simulink model "mixed_sensitivity_nonlin"  (R2022b)
settings: Solver=VariableStepAuto  StartTime=0.0  StopTime=1000  RelTol=1e-3
values from neighbouring files (symbols this model uses):
  a = Mv+mp+2*ma+2*IAy/(ra^2)    (= 19.1666666667)    [function_f.m]
  b = 1/2*(Mv*l^2+mp*L^2+2*ma*d^2+IGz+IPz+2*IAz+2*IAy*(d/ra)^2)    (= 3.3525)    [function_f.m]
  IPy = 0.15    [function_f.m]
  IPz = 0.23    [function_f.m]
  L = 1    [function_f.m]
  rp = 0.3    [function_f.m]
undefined symbols (not defined in the file or in its folder): Amix, Bmix, Cmix, Dmix, X_start_lqg_nonlin
settings Model: Creator=franc  LastModifiedBy=Giorgia

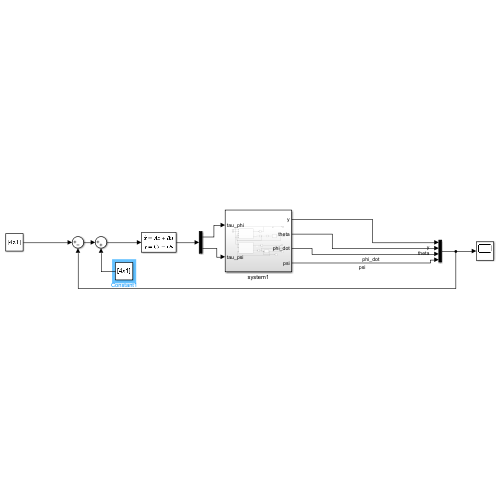
[thumbnail: Simulink's stored preview of the top-level diagram]
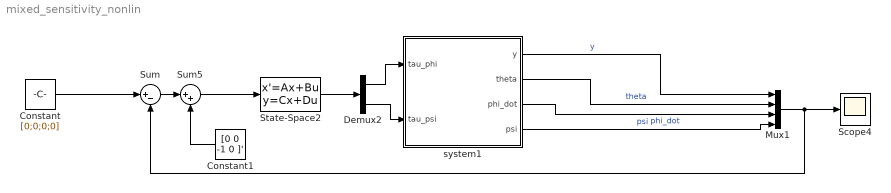
== system mixed_sensitivity_nonlin ==
  Constant : Constant  Value=[0;0;0;0]
  Constant1 : Constant  Value=[0 0 -1 0 ]'
  Demux2 : Demux  Outputs=2
  Mux1 : Mux
  Scope4 : Scope
  State-Space2 : StateSpace  A=Amix  B=Bmix  C=Cmix  D=Dmix  InitialCondition=0  ParameterTunability=Unconstrained
  Sum : Sum  Inputs=|+-
  Sum5 : Sum  Inputs=|++
  system1 : Subsystem
  wires:
  Constant/1 -> Sum/1
  State-Space2/1 -> Demux2/1
  Demux2/2 -> system1/2(tau_psi)
  Demux2/1 -> system1/1(tau_phi)
  system1/4(psi) -> Mux1/4  "psi"
  system1/3(phi_dot) -> Mux1/3  "phi_dot"
  system1/2(theta) -> Mux1/2  "theta"
  system1/1(y) -> Mux1/1  "y"
  Mux1/1 -> Sum/2, Scope4/1
  Sum/1 -> Sum5/1
  Sum5/1 -> State-Space2/1
  Constant1/1 -> Sum5/2

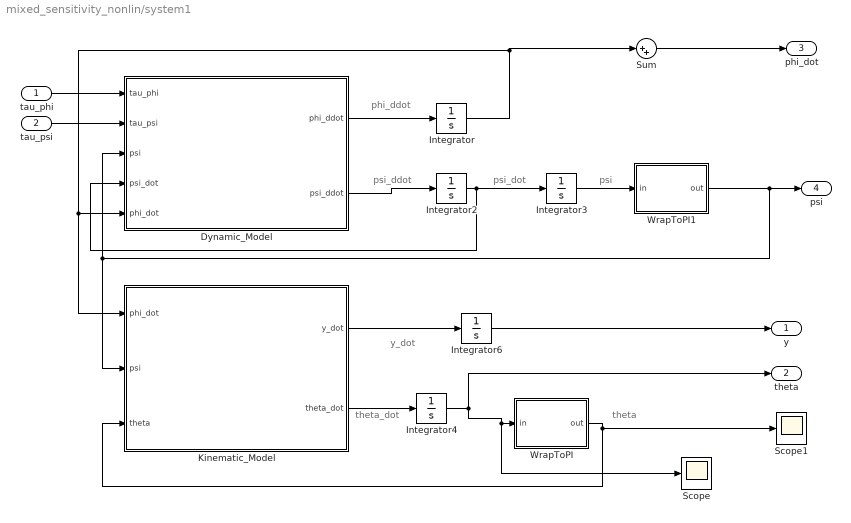
== system mixed_sensitivity_nonlin/system1 ==
  note: theta_dot
  note: psi_dot
  note: psi_ddot
  note: phi_ddot
  note: psi
  note: theta
  note: y_dot
  tau_phi : Inport
  tau_psi : Inport  Port=2
  Dynamic_Model : MATLAB Function  TreatAsAtomicUnit=on
  Integrator : Integrator  InitialCondition=X_start_lqg_nonlin(3)
  Integrator2 : Integrator  InitialCondition=X_start_lqg_nonlin(5)
  Integrator3 : Integrator  InitialCondition=X_start_lqg_nonlin(4)
  Integrator4 : Integrator  InitialCondition=X_start_lqg_nonlin(2)
  Integrator6 : Integrator  InitialCondition=X_start_lqg_nonlin(1)
  Kinematic_Model : MATLAB Function  TreatAsAtomicUnit=on
  Scope : Scope
  Scope1 : Scope
  Sum : Sum  Inputs=|++
  WrapToPI : MATLAB Function  TreatAsAtomicUnit=on
  WrapToPI1 : MATLAB Function  TreatAsAtomicUnit=on
  y : Outport
  theta : Outport  Port=2
  phi_dot : Outport  Port=3
  psi : Outport  Port=4
  wires:
  Integrator6/1 -> y/1
  WrapToPI1/1(out) -> psi/1, Dynamic_Model/3(psi), Kinematic_Model/2(psi)
  Integrator2/1 -> Integrator3/1, Dynamic_Model/4(psi_dot)
  tau_phi/1 -> Dynamic_Model/1(tau_phi)
  Integrator3/1 -> WrapToPI1/1(in)
  Integrator4/1 -> Scope/1, WrapToPI/1(in), theta/1
  Integrator/1 -> Kinematic_Model/1(phi_dot), Dynamic_Model/5(phi_dot), Sum/1
  Kinematic_Model/1(y_dot) -> Integrator6/1
  Kinematic_Model/2(theta_dot) -> Integrator4/1
  Dynamic_Model/2(psi_ddot) -> Integrator2/1
  Dynamic_Model/1(phi_ddot) -> Integrator/1
  WrapToPI/1(out) -> Kinematic_Model/3(theta), Scope1/1
  tau_psi/1 -> Dynamic_Model/2(tau_psi)
  Sum/1 -> phi_dot/1

== matlab function mixed_sensitivity_nonlin/system1/Dynamic_Model ==
  data: tau_phi input; tau_psi input; phi_ddot output; psi input; psi_dot input; phi_dot input; psi_ddot output; IPz parameter; IPy parameter; L parameter; rp parameter; b parameter; a parameter
function [phi_ddot,psi_ddot] = DynamicModel(tau_phi,tau_psi,psi,psi_dot,phi_dot,IPz, IPy, L, rp, b, a)
    B = [a*rp^2*cos(psi)^2+b*(rp/L)^2*sin(psi)^2+IPy, -IPz*(rp/L)*sin(psi)
        -IPz*(rp/L)*sin(psi), IPz];
    
    C = [(rp^2*b/L^2-a*rp^2)*cos(psi)*sin(psi)*psi_dot*phi_dot;
            -IPz*rp/L*cos(psi)*psi_dot*phi_dot];

    tau = [tau_phi;
            tau_psi];

    q_ddot = inv(B) * (tau - C);

    phi_ddot = q_ddot(1,:);
    psi_ddot = q_ddot(2,:);

== matlab function mixed_sensitivity_nonlin/system1/Kinematic_Model ==
  data: phi_dot input; psi input; theta input; y_dot output; theta_dot output; rp parameter; L parameter
function [y_dot,theta_dot] = KinematicModel(phi_dot,psi,theta,rp, L)
    x_dot = rp * phi_dot * cos(theta) * cos(psi);
    y_dot = rp * phi_dot * sin(theta) * cos(psi);
    theta_dot = - (rp * phi_dot * sin(psi)) / L;

== matlab function mixed_sensitivity_nonlin/system1/WrapToPI ==
  data: in input; out output
function out = wrapper(in)
    out = wrapTo2Pi(in);

== matlab function mixed_sensitivity_nonlin/system1/WrapToPI1 ==
  data: in input; out output
function out = wrapper(in)
    out = wrapToPi(in);
